simulink model "Zeros"  (R2018a)
settings: Solver=VariableStepAuto  StartTime=0.0  StopTime=10.0  RelTol=1e-3
values from neighbouring files (symbols this model uses):
  B = 20e3    (= 20000)    [LAB2.m]
  j = 600e3    (= 600000)    [LAB2.m]
  k = 2000    [LAB2.m]
settings Model: Creator=Ahmed Eldokmak  LastModifiedBy=Ahmed Eldokmak

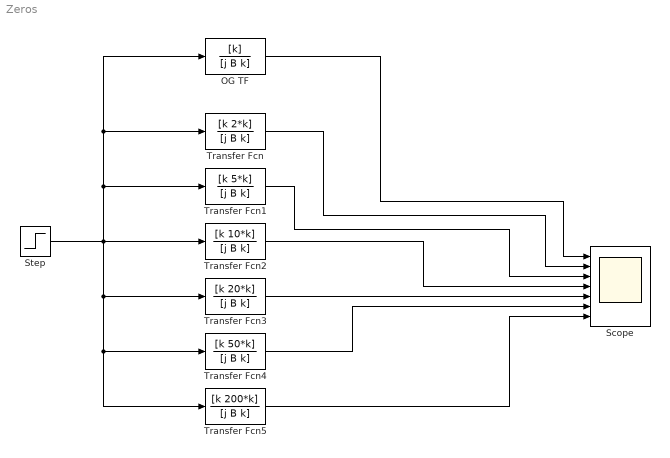
== system Zeros ==
  OG TF : TransferFcn  Numerator=[k]  Denominator=[j B k]
  Scope : Scope  NumInputPorts=7
  Step : Step  SampleTime=0
  Transfer Fcn : TransferFcn  Numerator=[k 2*k]  Denominator=[j B k]
  Transfer Fcn1 : TransferFcn  Numerator=[k 5*k]  Denominator=[j B k]
  Transfer Fcn2 : TransferFcn  Numerator=[k 10*k]  Denominator=[j B k]
  Transfer Fcn3 : TransferFcn  Numerator=[k 20*k]  Denominator=[j B k]
  Transfer Fcn4 : TransferFcn  Numerator=[k 50*k]  Denominator=[j B k]
  Transfer Fcn5 : TransferFcn  Numerator=[k 200*k]  Denominator=[j B k]
  wires:
  Step/1 -> Transfer Fcn5/1, Transfer Fcn4/1, Transfer Fcn3/1, Transfer Fcn1/1, Transfer Fcn/1, OG TF/1, Transfer Fcn2/1
  OG TF/1 -> Scope/1
  Transfer Fcn/1 -> Scope/2
  Transfer Fcn1/1 -> Scope/3
  Transfer Fcn2/1 -> Scope/4
  Transfer Fcn3/1 -> Scope/5
  Transfer Fcn4/1 -> Scope/6
  Transfer Fcn5/1 -> Scope/7
